simulink model "Modeliranje_i_upravljanje_letjelicom_diskretna_verzija"  (R2020b)
settings: Solver=VariableStepAuto  StartTime=0.0  StopTime=10  RelTol=1e-3
undefined symbols (not defined in the file): k_p2, k_r2, k_y2, k_z, wn_p2, wn_r2, wn_y2, wn_z, zeta_p2, zeta_r2, zeta_y2
settings Model: Creator=robert  LastModifiedBy=Ivan
settings SolverCC: ZeroCrossAlgorithm=Adaptive
settings DebuggingCC: IgnoredZcDiagnostic=none

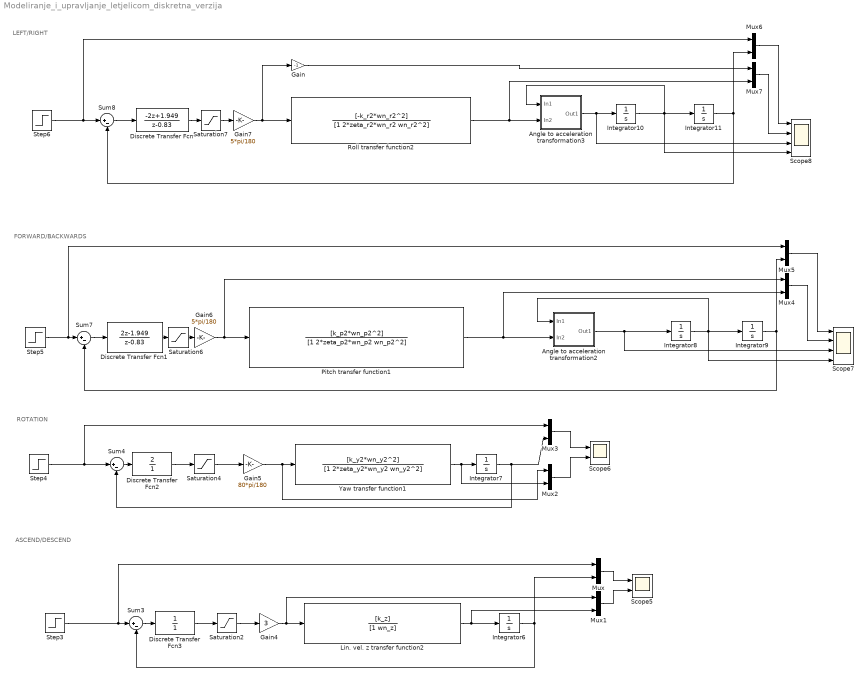
== system Modeliranje_i_upravljanje_letjelicom_diskretna_verzija ==
  note: ASCEND/DESCEND
  note: ROTATION
  note: FORWARD/BACKWARDS
  note: LEFT/RIGHT
  Angle to acceleration transformation2 : Subsystem
  Angle to acceleration transformation3 : Subsystem
  Discrete Transfer Fcn : DiscreteTransferFcn  Numerator=[-2 1.949]  Denominator=[1 -0.83]  SampleTime=0.1
  Discrete Transfer Fcn1 : DiscreteTransferFcn  Numerator=[2 -1.949]  Denominator=[1 -0.83]  SampleTime=0.1
  Discrete Transfer Fcn2 : DiscreteTransferFcn  Numerator=[2]  Denominator=[1]  SampleTime=0.1
  Discrete Transfer Fcn3 : DiscreteTransferFcn  Denominator=[1]  SampleTime=0.1
  Gain : Gain  Gain=-1
  Gain4 : Gain  Gain=3
  Gain5 : Gain  Gain=80*pi/180
  Gain6 : Gain  Gain=5*pi/180
  Gain7 : Gain  Gain=5*pi/180
  Integrator{6..11} (6 alike) : Integrator
  Lin. vel. z transfer function2 : TransferFcn  Numerator=[k_z]  Denominator=[1 wn_z]
  Mux{,1..7} (8 alike) : Mux  Inputs=2
  Pitch transfer function1 : TransferFcn  Numerator=[k_p2*wn_p2^2]  Denominator=[1 2*zeta_p2*wn_p2 wn_p2^2]
  Roll transfer function2 : TransferFcn  Numerator=[-k_r2*wn_r2^2]  Denominator=[1 2*zeta_r2*wn_r2 wn_r2^2]
  Saturation{2,4,6..7} (4 alike) : Saturate  UpperLimit=1  LowerLimit=-1
  Scope5 : Scope  NumInputPorts=2
  Scope6 : Scope  NumInputPorts=2
  Scope7 : Scope  NumInputPorts=4
  Scope8 : Scope  NumInputPorts=4
  Step3 : Step  Time=0  SampleTime=0
  Step4 : Step  Time=0  After=pi/4  SampleTime=0
  Step5 : Step  Time=0  After=2  SampleTime=0
  Step6 : Step  Time=0  After=2  SampleTime=0
  Sum{3..4,7..8} (4 alike) : Sum  Inputs=|+-
  Yaw transfer function1 : TransferFcn  Numerator=[k_y2*wn_y2^2]  Denominator=[1 2*zeta_y2*wn_y2 wn_y2^2]
  wires:
  Gain4/1 -> Mux1/1, Lin. vel. z transfer function2/1
  Saturation2/1 -> Gain4/1
  Step3/1 -> Mux/1, Sum3/1
  Integrator6/1 -> Mux/2, Sum3/2
  Lin. vel. z transfer function2/1 -> Mux1/2, Integrator6/1
  Gain5/1 -> Mux2/1, Yaw transfer function1/1
  Step4/1 -> Mux3/1, Sum4/1
  Saturation4/1 -> Gain5/1
  Integrator7/1 -> Sum4/2, Mux3/2
  Yaw transfer function1/1 -> Mux2/2, Integrator7/1
  Gain6/1 -> Mux4/1, Pitch transfer function1/1
  Step5/1 -> Mux5/1, Sum7/1
  Angle to acceleration transformation2/1(Out1) -> Scope7/3, Integrator8/1
  Integrator8/1 -> Angle to acceleration transformation2/1(In1), Scope7/4, Integrator9/1
  Saturation6/1 -> Gain6/1
  Pitch transfer function1/1 -> Mux4/2, Angle to acceleration transformation2/2(In2)
  Integrator9/1 -> Mux5/2, Sum7/2
  Gain7/1 -> Gain/1, Roll transfer function2/1
  Integrator11/1 -> Mux6/2, Sum8/2
  Integrator10/1 -> Angle to acceleration transformation3/1(In1), Scope8/4, Integrator11/1
  Angle to acceleration transformation3/1(Out1) -> Scope8/3, Integrator10/1
  Roll transfer function2/1 -> Mux7/2, Angle to acceleration transformation3/2(In2)
  Saturation7/1 -> Gain7/1
  Step6/1 -> Mux6/1, Sum8/1
  Mux1/1 -> Scope5/2
  Mux/1 -> Scope5/1
  Mux2/1 -> Scope6/2
  Mux3/1 -> Scope6/1
  Mux5/1 -> Scope7/1
  Mux4/1 -> Scope7/2
  Mux6/1 -> Scope8/1
  Mux7/1 -> Scope8/2
  Discrete Transfer Fcn/1 -> Saturation7/1
  Sum8/1 -> Discrete Transfer Fcn/1
  Sum7/1 -> Discrete Transfer Fcn1/1
  Discrete Transfer Fcn1/1 -> Saturation6/1
  Sum4/1 -> Discrete Transfer Fcn2/1
  Discrete Transfer Fcn2/1 -> Saturation4/1
  Sum3/1 -> Discrete Transfer Fcn3/1
  Discrete Transfer Fcn3/1 -> Saturation2/1
  Gain/1 -> Mux7/1

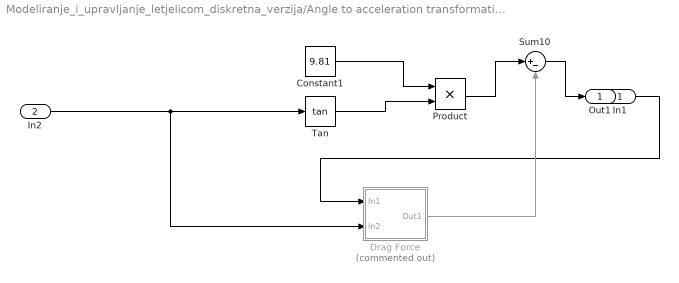
== system Modeliranje_i_upravljanje_letjelicom_diskretna_verzija/Angle to acceleration transformation2 ==
  In1 : Inport
  In2 : Inport  Port=2
  Constant1 : Constant  Value=9.81
  Drag Force : Subsystem  Commented=on
  Product : Product
  Sum10 : Sum  Inputs=|+-
  Tan : Trigonometry  Operator=tan
  Out1 : Outport
  wires:
  In2/1 -> Drag Force/2(In2), Tan/1
  Sum10/1 -> Out1/1
  Product/1 -> Sum10/1
  Tan/1 -> Product/2
  Constant1/1 -> Product/1
  In1/1 -> Drag Force/1(In1)
  Drag Force/1(Out1) -> Sum10/2

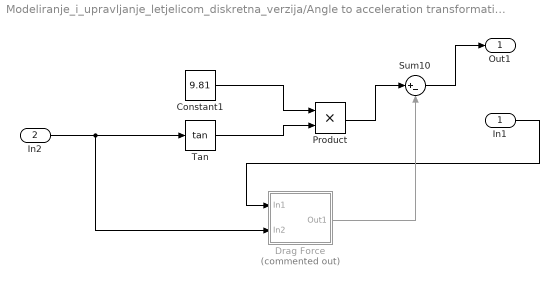
== system Modeliranje_i_upravljanje_letjelicom_diskretna_verzija/Angle to acceleration transformation3 ==
  In1 : Inport
  In2 : Inport  Port=2
  Constant1 : Constant  Value=9.81
  Drag Force : Subsystem  Commented=on
  Product : Product
  Sum10 : Sum  Inputs=|+-
  Tan : Trigonometry  Operator=tan
  Out1 : Outport
  wires:
  In2/1 -> Drag Force/2(In2), Tan/1
  Constant1/1 -> Product/1
  Tan/1 -> Product/2
  Product/1 -> Sum10/1
  Sum10/1 -> Out1/1
  In1/1 -> Drag Force/1(In1)
  Drag Force/1(Out1) -> Sum10/2

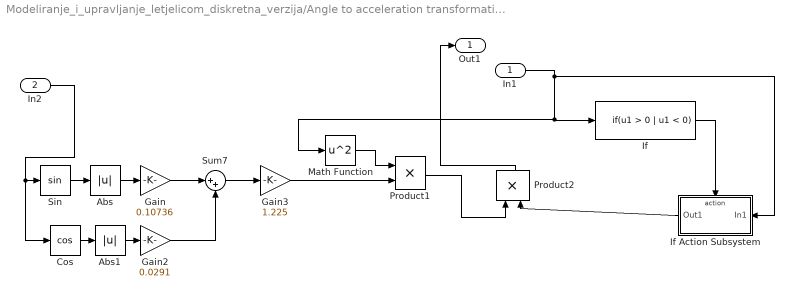
== system Modeliranje_i_upravljanje_letjelicom_diskretna_verzija/Angle to acceleration transformation2/Drag Force ==
  In1 : Inport
  In2 : Inport  Port=2
  Abs : Abs
  Abs1 : Abs
  Cos : Trigonometry  Operator=cos
  Gain : Gain  Gain=0.10736
  Gain2 : Gain  Gain=0.0291
  Gain3 : Gain  Gain=1.225
  If : If  IfExpression=u1 > 0 | u1 < 0  ShowElse=off
  If Action Subsystem : Subsystem  TreatAsAtomicUnit=on
  Math Function : Math  Operator=square  SaturateOnIntegerOverflow=on
  Product1 : Product
  Product2 : Product
  Sin : Trigonometry
  Sum7 : Sum  Inputs=|++
  Out1 : Outport
  wires:
  Cos/1 -> Abs1/1
  Abs/1 -> Gain/1
  Sum7/1 -> Gain3/1
  In1/1 -> If/1, Math Function/1, If Action Subsystem/1(In1)
  If Action Subsystem/1(Out1) -> Product2/2
  Sin/1 -> Abs/1
  In2/1 -> Sin/1, Cos/1
  Gain2/1 -> Sum7/2
  Math Function/1 -> Product1/1
  Abs1/1 -> Gain2/1
  Product1/1 -> Product2/1
  If/1 -> If Action Subsystem/Action
  Gain3/1 -> Product1/2
  Gain/1 -> Sum7/1
  Product2/1 -> Out1/1

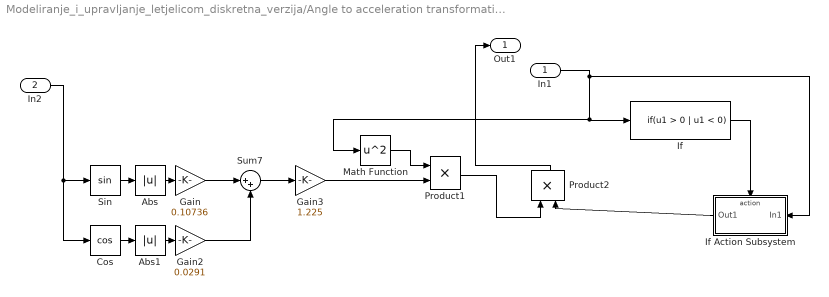
== system Modeliranje_i_upravljanje_letjelicom_diskretna_verzija/Angle to acceleration transformation3/Drag Force ==
  In1 : Inport
  In2 : Inport  Port=2
  Abs : Abs
  Abs1 : Abs
  Cos : Trigonometry  Operator=cos
  Gain : Gain  Gain=0.10736
  Gain2 : Gain  Gain=0.0291
  Gain3 : Gain  Gain=1.225
  If : If  IfExpression=u1 > 0 | u1 < 0  ShowElse=off
  If Action Subsystem : Subsystem  TreatAsAtomicUnit=on
  Math Function : Math  Operator=square  SaturateOnIntegerOverflow=on
  Product1 : Product
  Product2 : Product
  Sin : Trigonometry
  Sum7 : Sum  Inputs=|++
  Out1 : Outport
  wires:
  In1/1 -> If Action Subsystem/1(In1), Math Function/1, If/1
  Cos/1 -> Abs1/1
  Gain3/1 -> Product1/2
  Product2/1 -> Out1/1
  Sum7/1 -> Gain3/1
  In2/1 -> Sin/1, Cos/1
  Abs1/1 -> Gain2/1
  Gain2/1 -> Sum7/2
  Math Function/1 -> Product1/1
  Sin/1 -> Abs/1
  Product1/1 -> Product2/1
  Gain/1 -> Sum7/1
  Abs/1 -> Gain/1
  If/1 -> If Action Subsystem/Action
  If Action Subsystem/1(Out1) -> Product2/2

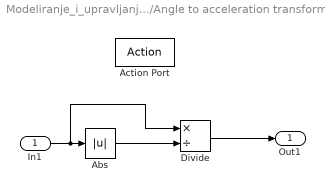
== system Modeliranje_i_upravljanje_letjelicom_diskretna_verzija/Angle to acceleration transformation2/Drag Force/If Action Subsystem ==
  In1 : Inport
  Action Port : ActionPort  ActionPortLabel=if(u1 > 0 | u1 < 0)
  Abs : Abs
  Divide : Product  Inputs=*/
  Out1 : Outport
  wires:
  Divide/1 -> Out1/1
  In1/1 -> Abs/1, Divide/1
  Abs/1 -> Divide/2

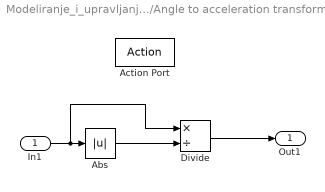
== system Modeliranje_i_upravljanje_letjelicom_diskretna_verzija/Angle to acceleration transformation3/Drag Force/If Action Subsystem ==
  In1 : Inport
  Action Port : ActionPort  ActionPortLabel=if(u1 > 0 | u1 < 0)
  Abs : Abs
  Divide : Product  Inputs=*/
  Out1 : Outport
  wires:
  Abs/1 -> Divide/2
  In1/1 -> Divide/1, Abs/1
  Divide/1 -> Out1/1
